simulink model "Lab1A_C3"  (R2019b)
settings: Solver=VariableStepAuto  StartTime=0.0  StopTime=10.0  RelTol=1e-3
settings Model: Creator=sinow  LastModifiedBy=sinow

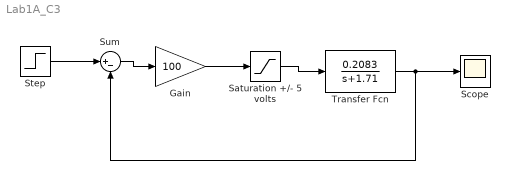
== system Lab1A_C3 ==
  Gain : Gain  Gain=100
  Saturation +/- 5 volts : Saturate  UpperLimit=5  LowerLimit=-5
  Scope : Scope
  Step : Step  Time=0  After=10  SampleTime=0
  Sum : Sum  Inputs=|+-
  Transfer Fcn : TransferFcn  Numerator=0.2083  Denominator=[1 1.71]
  wires:
  Step/1 -> Sum/1
  Sum/1 -> Gain/1
  Gain/1 -> Saturation +/- 5 volts/1
  Saturation +/- 5 volts/1 -> Transfer Fcn/1
  Transfer Fcn/1 -> Sum/2, Scope/1
